simulink model "oscillator"  (Simulink 10.0)
settings: Solver=VariableStepAuto  StartTime=0.0  StopTime=20.0  RelTol=1e-3
values from neighbouring files (symbols this model uses):
  C = [1 1]    [ChemReactor.m]    (also in MagLevit.m = [1 0]; TF.m = [-0.2 0]; final-constants.m = 0.25; final-problem1.m = 0.25)
  L = 0.229    [MagLevit.m]    (also in final-constants.m = 1.6; final-problem1.m = 1.6)
  R1 = 4    [final-constants.m]    (also in final-problem1.m)
  R2 = 2    [final-constants.m]    (also in final-estimate_price.m = 1-(SSE/SST); final-problem1.m; problem3.m = 1-(SSE/SST))
  R3 = 3    [final-constants.m]    (also in final-problem1.m)
settings Model: Creator=aravind  LastModifiedBy=aravind
settings DataIOCC: SaveFormat=Dataset  ReturnWorkspaceOutputs=on
settings OptimizationCC: LifeSpan=auto
settings DebuggingCC: UnderspecifiedInitializationDetection=Simplified  MergeDetectMultiDrivingBlocksExec=error  SFUnexpectedBacktrackingDiag=error  SFNoUnconditionalDefaultTransitionDiag=error  SFExecutionAtInitializationDiag=warning  ArithmeticOperatorsInVariantConditions=error
settings HardwareCC: ProdBitPerPointer=64  ProdBitPerSizeT=64  ProdBitPerPtrDiffT=64  ProdLargestAtomicFloat=Float  ProdIntDivRoundTo=Zero  ProdEndianess=LittleEndian  ProdWordSize=64  ProdHWDeviceType=Intel->x86-64 (Windows64)
settings ModelReferenceCC: PropagateSignalLabelsOutOfModel=on
settings SFSimCC: SimUseLocalCustomCode=on  CustomCodeUndefinedFunction=FilterOut
settings RTWCC: RTWUseLocalCustomCode=on
settings CodeAppCC: StateflowObjectComments=off
settings GRTTargetCC: TargetLangStandard=C99 (ISO)  CombineOutputUpdateFcns=on  GRTInterface=off
settings ConfigComp: CovMetricSettings=dwe  CovHtmlReporting=off  CovSaveCumulativeToWorkspaceVar=off  CovSaveSingleToWorkspaceVar=off

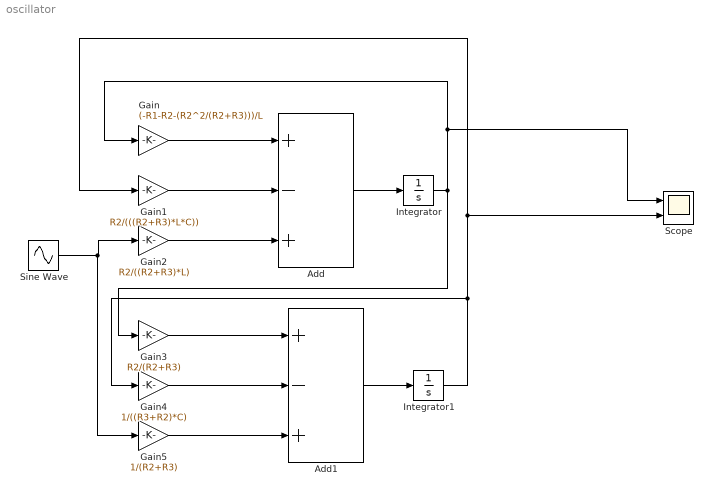
== system oscillator ==
  Add : Sum  Inputs=+-+
  Add1 : Sum  Inputs=+-+
  Gain : Gain  Gain=(-R1-R2-(R2^2/(R2+R3)))/L
  Gain1 : Gain  Gain=R2/(((R2+R3)*L*C))
  Gain2 : Gain  Gain=R2/((R2+R3)*L)
  Gain3 : Gain  Gain=R2/(R2+R3)
  Gain4 : Gain  Gain=1/((R3+R2)*C)
  Gain5 : Gain  Gain=1/(R2+R3)
  Integrator : Integrator  InitialCondition=15
  Integrator1 : Integrator  InitialCondition=2
  Scope : Scope  NumInputPorts=2
  Sine Wave : Sin  SampleTime=0
  wires:
  Add/1 -> Integrator/1
  Gain/1 -> Add/1
  Gain1/1 -> Add/2
  Gain2/1 -> Add/3
  Sine Wave/1 -> Gain5/1, Gain2/1
  Add1/1 -> Integrator1/1
  Gain3/1 -> Add1/1
  Gain4/1 -> Add1/2
  Gain5/1 -> Add1/3
  Integrator1/1 -> Gain4/1, Scope/2, Gain1/1
  Integrator/1 -> Gain3/1, Gain/1, Scope/1
